simulink model "LQControlReducedOrderObserver"  (R2015a)
settings: Solver=ode45  StartTime=0.0  StopTime=tijd  RelTol=1e-3
values from neighbouring files (symbols this model uses):
  A2 = A    [LQControl.m]    (also in LQControl_script.m)
  AR = AT2(1,1) - HR*AT2(2:3,1)    [LQControl.m]    (also in LQControl_script.m)
  B2 = B    [LQControl.m]    (also in LQControl_script.m)
  BR = [(AT2(1,1)-HR*AT2(2:3,1))*HR + AT2(1,2:3)-HR*AT2(2:3,2:3) BT2(1)-HR*BT2(2:3) - (AT2(1,1)-HR*AT2(2:3,1))*HR*D2]    [LQControl.m]    (also in LQControl_script.m)
  C2 = [0.5 0.4 0 ... (first row only)    [LQControl.m]    (also in LQControl_script.m)
  CR = 1    [LQControl.m]    (also in LQControl_script.m)
  D2 = [0;0]    [LQControl.m]    (also in LQControl_script.m)
  DR = [0 0 0]    [LQControl.m]    (also in LQControl_script.m)
  HR = [-22.75 0]    [LQControl.m]    (also in LQControl_script.m)
  init = 0 - HR*C2*[k0-kev;s0;v0-vev] + HR * D2 * kin    [LQControl.m]    (also in LQControl_script.m)
  k0 = -1.22*10^3    (= -1220)    [LQControl.m]    (also in LQControl_script.m)
  kev = (Y*a*kV)/(d1 - b1 + Y*a)    (= 2222.22222222)    [LQControl.m]    (also in LQControl_script.m)
  kin = 0    [LQControl.m]    (also in LQControl_script.m)
  s0 = 500    [LQControl.m]    (also in LQControl_script.m)
  TR = [1 0 0;C2]    [LQControl.m]    (also in LQControl_script.m)
  v0 = -2.22    [LQControl.m]    (also in LQControl_script.m)
  vev = (a*kV*(b1 - d1))/(d3*(d1 - b1 + Y*a))    (= 22.2222222222)    [LQControl.m]    (also in LQControl_script.m)
settings Model: Creator=Ward  LastModifiedBy=Ward

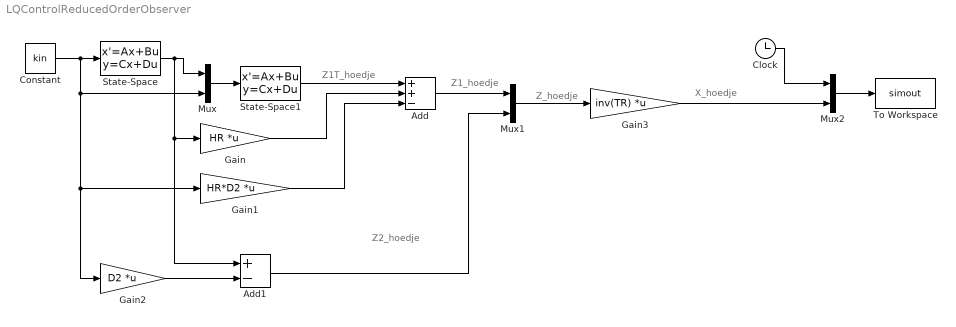
== system LQControlReducedOrderObserver ==
  note: X_hoedje
  note: Z_hoedje
  note: Z2_hoedje
  note: Z1_hoedje
  note: Z1T_hoedje
  Add : Sum  Inputs=++-
  Add1 : Sum  Inputs=+-
  Clock : Clock
  Constant : Constant  Value=kin
  Gain : Gain  Gain=HR  Multiplication=Matrix(K*u)
  Gain1 : Gain  Gain=HR*D2  Multiplication=Matrix(K*u)
  Gain2 : Gain  Gain=D2  Multiplication=Matrix(K*u)
  Gain3 : Gain  Gain=inv(TR)  Multiplication=Matrix(K*u)
  Mux : Mux  Inputs=2
  Mux1 : Mux  Inputs=2
  Mux2 : Mux  Inputs=2
  State-Space : StateSpace  A=A2  B=B2  C=C2  D=D2  X0=[k0-kev;s0;v0-vev]
  State-Space1 : StateSpace  A=AR  B=BR  C=CR  D=DR  X0=init
  To Workspace : ToWorkspace  VariableName=simout  SampleTime=-1
  wires:
  Constant/1 -> Gain2/1, Gain1/1, Mux/2, State-Space/1
  Clock/1 -> Mux2/1
  Mux/1 -> State-Space1/1
  State-Space/1 -> Add1/1, Gain/1, Mux/1
  State-Space1/1 -> Add/1
  Gain/1 -> Add/2
  Gain1/1 -> Add/3
  Add/1 -> Mux1/1
  Mux1/1 -> Gain3/1
  Mux2/1 -> To Workspace/1
  Gain3/1 -> Mux2/2
  Gain2/1 -> Add1/2
  Add1/1 -> Mux1/2
